simulink model "Propofol_OL_2023"  (R2023a)
settings: Solver=VariableStepAuto  StartTime=0.0  StopTime=100  RelTol=1e-3
values from neighbouring files (symbols this model uses):
  delay = Patient(patient, 1)    [PlotME.m]
  E0 = Patient(patient, 5)    [PlotME.m]
  E50 = Patient(patient, 3)    [PlotME.m]
  gamma = Patient(patient, 4)    [PlotME.m]
  k = Patient(patient, 2)    [PlotME.m]
settings Model: Creator=mluser  LastModifiedBy=Gabriel
settings SolverCC: AlgebraicLoopSolver=TrustRegion
settings DebuggingCC: ArithmeticOperatorsInVariantConditions=warning
settings ModelReferenceCC: EnableRefExpFcnMdlSchedulingChecks=on
settings SFSimCC: CustomCodeUndefinedFunction=UseInterfaceOnly
settings CodeAppCC: StateflowObjectComments=on

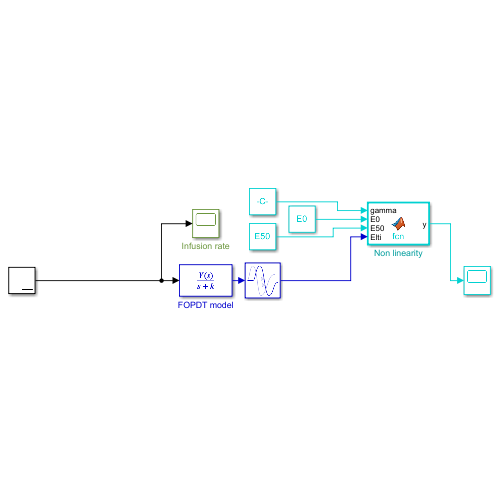
[thumbnail: Simulink's stored preview of the top-level diagram]
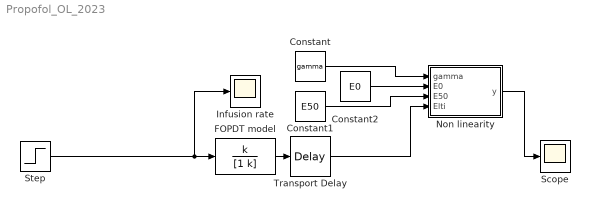
== system Propofol_OL_2023 ==
  Constant : Constant  Value=gamma
  Constant1 : Constant  Value=E50
  Constant2 : Constant  Value=E0
  FOPDT model : TransferFcn  Numerator=k  Denominator=[1 k]
  Infusion rate : Scope
  Non linearity : MATLAB Function  TreatAsAtomicUnit=on
  Scope : Scope
  Step : Step  Before=E0  After=50  SampleTime=0
  Transport Delay : TransportDelay  DelayTime=delay/60
  wires:
  FOPDT model/1 -> Transport Delay/1
  Step/1 -> Infusion rate/1, FOPDT model/1
  Transport Delay/1 -> Non linearity/4(Elti)
  Constant/1 -> Non linearity/1(gamma)
  Constant1/1 -> Non linearity/3(E50)
  Constant2/1 -> Non linearity/2(E0)
  Non linearity/1(y) -> Scope/1

== matlab function Propofol_OL_2023/Non linearity ==
  data: gamma input; y output; E0 input; E50 input; Elti input
function y = fcn(gamma,E0,E50,Elti)

y = E0-E0*Elti^gamma/(E50^gamma+Elti^gamma);
